simulink model "task301"  (R2016a)
settings: Solver=VariableStepAuto  StartTime=0.0  StopTime=10.0  RelTol=1e-3
libraries: dspsrcs4 x2, simulink x1, dsparch4 x1
settings Model: Creator=Misachu  LastModifiedBy=Misachu

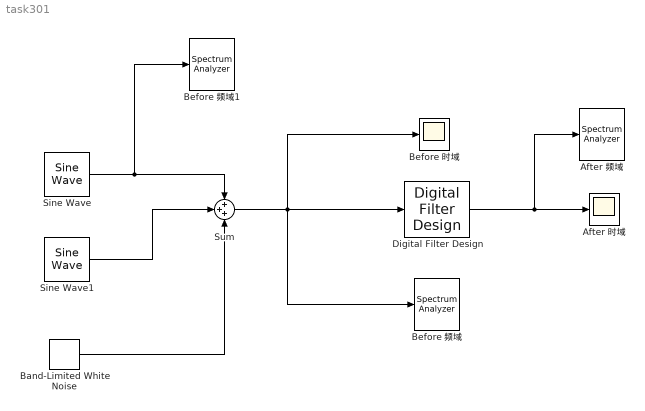
== system task301 ==
  After 时域 : Scope
  After 频域 : SpectrumAnalyzer
  Band-Limited White Noise : simulink/Sources/Band-Limited White Noise  Cov=[0.1]  Ts=0.1  seed=[23341]
  Before 时域 : Scope
  Before 频域 : SpectrumAnalyzer
  Before 频域1 : SpectrumAnalyzer
  Digital Filter Design : dsparch4/Digital Filter Design  mwdsp_browser_bugfix_var=off
  Sine Wave : dspsrcs4/Sine Wave  Amplitude=1  Frequency=300  Phase=0  SampleMode=Discrete  OutComplex=Real  CompMethod=Trigonometric fcn  TableSize=Speed  SampleTime=1/1000  SamplesPerFrame=1  ResetState=Restart at time zero  OutputFrames=off  dataType=double  wordLen=16  udDataType=sfix(16)  fracBitsMode=Best precision  numFracBits=15  OutDataTypeStr=double  LastOutDataTypeStr=double
  Sine Wave1 : dspsrcs4/Sine Wave  Amplitude=1  Frequency=100  Phase=0  SampleMode=Discrete  OutComplex=Real  CompMethod=Trigonometric fcn  TableSize=Speed  SampleTime=1/1000  SamplesPerFrame=1  ResetState=Restart at time zero  OutputFrames=off  dataType=double  wordLen=16  udDataType=sfix(16)  fracBitsMode=Best precision  numFracBits=15  OutDataTypeStr=double  LastOutDataTypeStr=double
  Sum : Sum  Inputs=3
  wires:
  Sine Wave/1 -> Before 频域1/1, Sum/1
  Sine Wave1/1 -> Sum/2
  Band-Limited White Noise/1 -> Sum/3
  Sum/1 -> Before 频域/1, Before 时域/1, Digital Filter Design/1
  Digital Filter Design/1 -> After 频域/1, After 时域/1
